simulink model "LINEARIZZAZIONE"  (R2022b)
settings: Solver=VariableStepAuto  StartTime=0.0  StopTime=10.0  RelTol=1e-3
libraries: simulink x1
settings Model: Creator=Utente  LastModifiedBy=Utente
settings OptimizationCC: BlockReduction=off  DefaultParameterBehavior=Inlined  BufferReuse=off

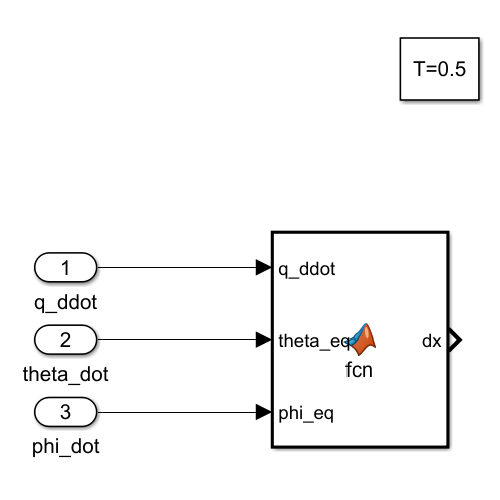
[thumbnail: Simulink's stored preview of the top-level diagram]
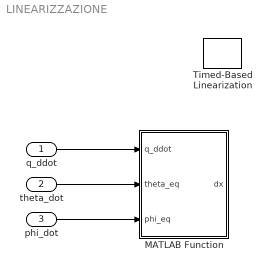
== system LINEARIZZAZIONE ==
  q_ddot : Inport
  theta_dot : Inport  Port=2
  phi_dot : Inport  Port=3
  MATLAB Function : MATLAB Function  TreatAsAtomicUnit=on
  Timed-Based Linearization : simulink/Model-Wide Utilities/Timed-Based Linearization  LinearizationTime=0.5  SampleTime=0
  wires:
  q_ddot/1 -> MATLAB Function/1(q_ddot)
  theta_dot/1 -> MATLAB Function/2(theta_eq)
  phi_dot/1 -> MATLAB Function/3(phi_eq)

== matlab function LINEARIZZAZIONE/MATLAB Function ==
  data: q_ddot input; dx output; theta_eq input; phi_eq input
function dx = fcn(q_ddot, theta_eq, phi_eq)

x2= theta_dot;
x4= phi_dot;

dx(1)= x2;
dx(2)= q_ddot(1);
dx(3)= x4;
dx(4)= q_ddot(2);

dx = [dx(1) dx(2) dx(3) dx(4)]';
